simulink library "Simple_House_ISO_GroundModel"  (Simulink 8.2)
settings: Solver=ode45  StartTime=0.0  StopTime=10.0  RelTol=1e-3
libraries: carnot x6, simulink x1
settings Model: Creator=lena.frank  LastModifiedBy=drhf

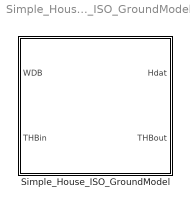
== system Simple_House_ISO_GroundModel ==
  Simple_House_ISO_GroundModel : Subsystem  mask(Simple House with ISO 13370 Ground Model){Ahabit=140, Hroom=2.6, Floorsize=[7 10], UAwall=0.162*(54.6+26.4)+0.182*((45.7+56.0)*2 -(12+4+3+4)), UAneighbour=0, Uground=0.1, mc=0.5e6*140 % 0.5 MJ/m2/K, shade=0.75, tini=20, Awin=[12 4 3 4], AziWin=[0 90 -180 -90], Uwin=[1    1   1    1]*1.0, Gwin=[1    1   1    1]*0.585*(1-0.15), vent=0.4, rec=0.6, heatload=1792, delta_t_nom=15, n_rad=1.1, mass_times_cap=40e6, dpcoeff=[10 100]}
      mask prompts: Ahabit "Living surface in m²"; Hroom "height of rooms in m"; Floorsize "Dimensions of slab in m [length width]"; UAwall "Total heat transfer to ambient (walls/roof) in W/K"; UAneighbour "Total heat transfer to neighbour inW/K"; Uground "Heat transfer coeffient of slab to ground in W/m²/K"; mc "Total thermal capacity in J/K"; shade "Shading factor [0..1] when T room > 4 K + T_init"; tini "Initial temperature"; Awin "Surface of 4 windows in m² (vector)"; AziWin "Orientation of 4 windows (south 0, east -90,west 90)"; Uwin "Heat loss coefficient 4 windows in W/m²/K [vector]"; Gwin "Light transmittance 4 windows (0..1) * (1 - frame_part) [vector]"; vent "Ventilation rate in 1/h"; rec "Heat recovery (0..1)"; heatload "Heating capacity radiator  [W]"; delta_t_nom "Nominal delta T (average radiator temperature - room temperature) [K]"; n_rad "Radiator exponent"; mass_times_cap "Mass*capacity of heating system [J/K]"; dpcoeff "Pressure drop coefficients [linear quadratic] in Pa/(kg/s), Pa/(kg/s)²"
      mask help:
      | Uses the simple model of 1-node room or house. The heating power is generated by a radiator or floor heating system.
      | The windows have an automatic shading (shading factor) if room temperature rises 4 K above initial temperature.
      | solar gain = Solar_Radiation_on_window * light_transmittance * shading_factor
      | The ground model of ISO 13370 is used to calculate the losses to the ground. Remember to set the values of the model according to the set point of the room temperature and the weather data.
      mask init:
      | invmc = 1/mc;
      | rec = max(0,min(1,rec));
      | Gwin = max(0,min(1,Gwin));
      | shade = max(0, min(1, shade));
      mask Help: web(fullfile(path_carnot('help'),'simple_house.html'),'-helpbrowser')
      mask Display:
      | plot(-20,-30,120,100,[10,10,90,90,10],[0,50,50,0,0],...
      |     [100,60,40,0],[40,80,80,40],[20,34,34,20,20],[40,40,20,20,40],...
      |     [60,60,40,40],[0,40,40,0],[65,80,80,65,65],[40,40,20,20,40],...
      |     [47,54,54,47,47],[35,35,4,4,35],[45,41],[20,20])

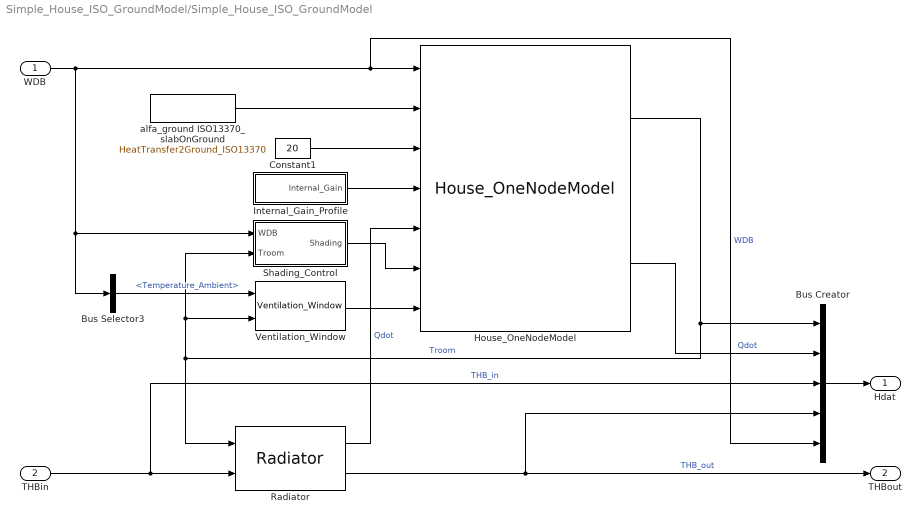
== system Simple_House_ISO_GroundModel/Simple_House_ISO_GroundModel ==
  WDB : Inport
  THBin : Inport  Port=2
  Bus Creator : BusCreator  Inputs=5
  Bus Selector3 : BusSelector  OutputSignals=Temperature_Ambient
  Constant1 : Constant  Value=20
  House_OneNodeModel : carnot/Basic/Thermal_Models/House_OneNodeModel  Ahabit=Ahabit  Hroom=Hroom  tini=tini  UAout=UAwall  mc=mc  UAin=UAneighbour  dtroom=inf  AziWin=AziWin  Awin=Awin  Uwin=Uwin  Gwin=Gwin
  Internal_Gain_Profile : Subsystem
  Radiator : carnot/Source/Heat_Exchanger/Radiator  pnom=heatload  dtnom=delta_t_nom  expo=n_rad  mcap=mass_times_cap  tini=tini  lin=0  qua=1000
  Shading_Control : Subsystem
  Ventilation_Window : carnot/Source/Ventilation/Ventilation_Window  vent=vent  rec=rec  Vhouse=Ahabit*Hroom
  alfa_ground ISO13370_slabOnGround : carnot/Load/Houses/heat_transfer/HeatTransfer2Ground_ISO13370  wallsize=Floorsize  gammat=0  Tmeaninside=23.8  deltathetai=3.8  Tmeanoutside=11  deltathetae=9.3  tshift=319*3600  dwall=0.4  cond_ground=2.0  cp_ground=800  rho_ground=2500  rtot=1/Uground
  Hdat : Outport
  THBout : Outport  Port=2
  wires:
  alfa_ground ISO13370_slabOnGround/1 -> House_OneNodeModel/2
  Bus Creator/1 -> Hdat/1
  Internal_Gain_Profile/1(Internal_Gain) -> House_OneNodeModel/4
  House_OneNodeModel/2 -> Bus Creator/2  "Qdot"
  Shading_Control/1(Shading) -> House_OneNodeModel/6
  House_OneNodeModel/1 -> Bus Creator/1, Radiator/1, Shading_Control/2(Troom), Ventilation_Window/2  "Troom"
  Bus Selector3/1 -> Ventilation_Window/1  "<Temperature_Ambient>"
  Radiator/1 -> House_OneNodeModel/5  "Qdot"
  Constant1/1 -> House_OneNodeModel/3
  Ventilation_Window/1 -> House_OneNodeModel/7
  Radiator/2 -> Bus Creator/4, THBout/1  "THB_out"
  THBin/1 -> Bus Creator/3, Radiator/2  "THB_in"
  WDB/1 -> House_OneNodeModel/1, Bus Creator/5, Shading_Control/1(WDB), Bus Selector3/1  "WDB"

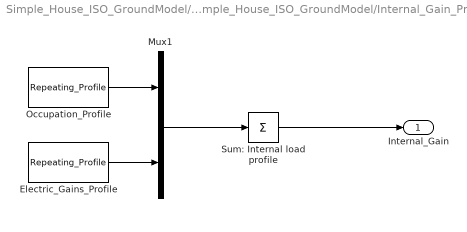
== system Simple_House_ISO_GroundModel/Simple_House_ISO_GroundModel/Internal_Gain_Profile ==
  Electric_Gains_Profile : carnot/Load/General/Repeating_Profile  period=24*3600  rep_seq_t=[0 1 6 7 8 9 11 12 13 18 19 20 22 23]*3600  rep_seq_d=[1 5 1 1 1 2 1 1 4 2 1 2 1 1]*3600  rep_seq_y=[105 55 392.5 457.5 420 55 250 55 120 170 615 420 442.5 355]
  Mux1 : Mux  Inputs=2
  Occupation_Profile : carnot/Load/General/Repeating_Profile  period=24*3600  rep_seq_t=[0 6 7 8 9 11 12 13 14 15 17 18 20 21 22]*3600  rep_seq_d=[6 1 1 1 2 1 1 1 1 2 1 2 1 1 2]*3600  rep_seq_y=[4 2 3 2 0 1 3 2 1 0 1 2 4 3 4]*60
  Sum: Internal load profile : Sum  Inputs=+
  Internal_Gain : Outport
  wires:
  Sum: Internal load profile/1 -> Internal_Gain/1
  Electric_Gains_Profile/1 -> Mux1/2
  Occupation_Profile/1 -> Mux1/1
  Mux1/1 -> Sum: Internal load profile/1

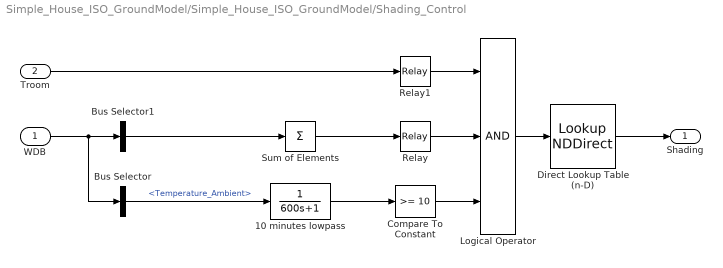
== system Simple_House_ISO_GroundModel/Simple_House_ISO_GroundModel/Shading_Control ==
  WDB : Inport
  Troom : Inport  Port=2
  10 minutes lowpass : TransferFcn  Denominator=[600 1]
  Bus Selector : BusSelector  OutputSignals=Temperature_Ambient
  Bus Selector1 : BusSelector  OutputSignals=Solar_Radiation_direct_surface,Solar_Radiation_diffuse_surface  OutputAsBus=on
  Compare To Constant : simulink/Logic and Bit Operations/Compare To Constant  relop=>=  const=10  OutDataTypeStr=uint8
  Direct Lookup Table (n-D) : LookupNDDirect  NumberOfTableDimensions=1  Table=[1 1-shade]
  Logical Operator : Logic  Inputs=3  AllPortsSameDT=off  OutDataTypeStr=boolean
  Relay : Relay  OnSwitchValue=300  OffSwitchValue=200  OutDataTypeStr=uint8
  Relay1 : Relay  OnSwitchValue=23.8  OffSwitchValue=22.8  OutDataTypeStr=uint8
  Sum of Elements : Sum  Inputs=+
  Shading : Outport
  wires:
  Bus Selector/1 -> 10 minutes lowpass/1  "<Temperature_Ambient>"
  Relay1/1 -> Logical Operator/1
  WDB/1 -> Bus Selector/1, Bus Selector1/1
  Direct Lookup Table (n-D)/1 -> Shading/1
  Troom/1 -> Relay1/1
  Compare To Constant/1 -> Logical Operator/3
  Relay/1 -> Logical Operator/2
  Sum of Elements/1 -> Relay/1
  Logical Operator/1 -> Direct Lookup Table (n-D)/1
  10 minutes lowpass/1 -> Compare To Constant/1
  Bus Selector1/1 -> Sum of Elements/1
